simulink model "Boost_Converter_22UEE051"  (R2023b)
settings: Solver=VariableStepAuto  StartTime=0.0  StopTime=3  RelTol=1e-3
libraries: spsVoltageMeasurementLib x5, spsCurrentMeasurementLib x4, spsSeriesRLCBranchLib x3, spsDCVoltageSourceLib x1, spsDiodeLib x1, spsMosfetLib x1, spspowerguiLib x1
settings Model: Creator=prita  LastModifiedBy=SWARUP
settings DebuggingCC: UnconnectedInputMsg=warning  UnconnectedOutputMsg=warning  UnconnectedLineMsg=warning
settings ModelReferenceCC: EnableRefExpFcnMdlSchedulingChecks=on
settings RTWCC: DLArmComputeVersion=19.05

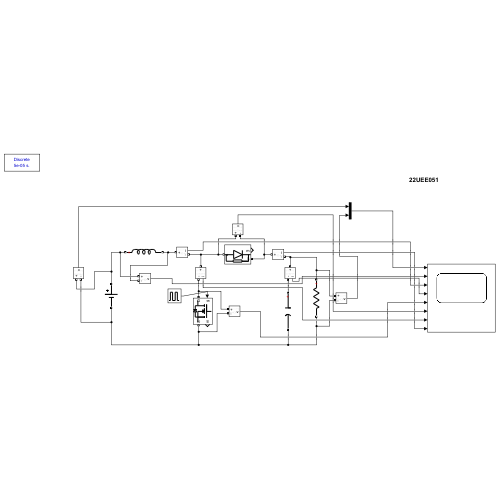
[thumbnail: Simulink's stored preview of the top-level diagram]
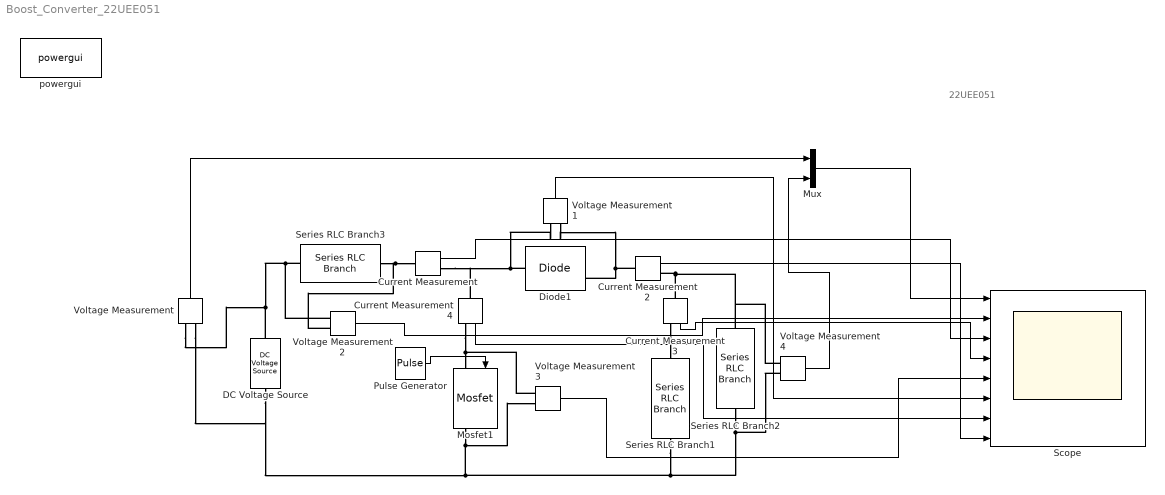
== system Boost_Converter_22UEE051 ==
  note: 22UEE051
  Current Measurement{,2..4} (4 alike) : spsCurrentMeasurementLib/Current Measurement  PhasorSimulation=off  OutputType=Complex  PSBequivalent=0
  DC Voltage Source : spsDCVoltageSourceLib/DC Voltage Source  Amplitude=12  Measurements=None
  Diode1 : spsDiodeLib/Diode  Ron=0.001  Lon=0  Vf=0  IC=0  UseSnubber=0  Rs=500  Cs=250e-9  Measurements=on
  Mosfet1 : spsMosfetLib/Mosfet  Ron=0.1  Lon=0  Rd=0.01  Vfd=0  IC=0  Rs=1e5  Cs=inf  Measurements=on
  Mux : Mux  Inputs=2
  Pulse Generator : DiscretePulseGenerator  PulseType=Time based  Period=0.02  PulseWidth=50
  Scope : Scope  NumInputPorts=8
  Series RLC Branch1 : spsSeriesRLCBranchLib/Series RLC Branch  LConnTagsString=__new0  RConnTagsString=__new0  BranchType=C  Resistance=1  Inductance=1e-3  SetiL0=off  InitialCurrent=0  Capacitance=0.2  Setx0=off  InitialVoltage=0  Measurements=None
  Series RLC Branch2 : spsSeriesRLCBranchLib/Series RLC Branch  LConnTagsString=__new0  RConnTagsString=__new0  BranchType=R  Resistance=10  Inductance=1e-3  SetiL0=off  InitialCurrent=0  Capacitance=1e-6  Setx0=off  InitialVoltage=0  Measurements=None
  Series RLC Branch3 : spsSeriesRLCBranchLib/Series RLC Branch  LConnTagsString=__new0  RConnTagsString=__new0  BranchType=L  Resistance=1  Inductance=15.625e-3  SetiL0=off  InitialCurrent=0  Capacitance=1e-6  Setx0=off  InitialVoltage=0  Measurements=None
  Voltage Measurement{,1..4} (5 alike) : spsVoltageMeasurementLib/Voltage Measurement  PhasorSimulation=off  OutputType=Complex  PSBequivalent=0
  powergui : spspowerguiLib/powergui  Priority=1  SimulationMode=Discrete  SampleTime=50e-6  frequency=60  Iterations=50  frequencyindice=0  Pbase=100e6  ErrMax=1e-4  UnitsV=kV  UnitsW=MW  buscounter=0  FunctionMessages=off  echomessages=off  EnableUseOfTLC=off  CurrentSourceSwitches=off  DisableSnubberDevices=off  DisableRonSwitches=off  DisableVfSwitches=off  DisplayEquations=off  AutomaticDiscreteSolvers=off  SolverType=Tustin/Backward Euler (TBE)  Interpol=off  ExternalGateDelay=off  methode=off  Ts=100  x0status=blocks  SPID=on  SwTol=0  HookPort=off  NonlinearTolerance=1e-4  nMaxIteration=100  ContinueOnMaxIteration=off  RestoreLinks=warning  ResistiveCurrentMeasurement=off  Frange=[0:2:500]  Ylog=off  Xlog=on  ShowGrid=off  save=off  variable=ZData  structure=0  ZoomFFT=off  StartTime=0.0  cycles=1  DisplayStyle=1  fundamental=60  FreqAxis=off  MaxFrequency=1000  frequencyindicesteady=1  RmsSteady=1  display=off
  wires:
  Voltage Measurement4/1 -> Mux/2
  Voltage Measurement/1 -> Mux/1
  Pulse Generator/1 -> Mosfet1/1
  Mux/1 -> Scope/1
  Voltage Measurement2/1 -> Scope/2
  Current Measurement/1 -> Scope/3
  Current Measurement3/1 -> Scope/4
  Voltage Measurement3/1 -> Scope/5
  Voltage Measurement1/1 -> Scope/6
  Current Measurement2/1 -> Scope/8
  Current Measurement4/1 -> Scope/7
  connections:
  Voltage Measurement2/LConn1 -- Series RLC Branch3/LConn1 -- DC Voltage Source/RConn1 -- Voltage Measurement/LConn1
  Series RLC Branch2/RConn1 -- DC Voltage Source/LConn1 -- Voltage Measurement/LConn2 -- Mosfet1/RConn1 -- Voltage Measurement3/LConn2 -- Series RLC Branch1/RConn1 -- Voltage Measurement4/LConn2
  Voltage Measurement3/LConn1 -- Current Measurement4/RConn1 -- Mosfet1/LConn1
  Current Measurement2/RConn1 -- Current Measurement3/LConn1 -- Voltage Measurement4/LConn1 -- Series RLC Branch2/LConn1
  Voltage Measurement1/LConn2 -- Diode1/RConn1 -- Current Measurement2/LConn1
  Voltage Measurement1/LConn1 -- Current Measurement4/LConn1 -- Current Measurement/RConn1 -- Diode1/LConn1
  Voltage Measurement2/LConn2 -- Series RLC Branch3/RConn1 -- Current Measurement/LConn1
  Current Measurement3/RConn1 -- Series RLC Branch1/LConn1
